simulink model "model2_smartDecision"  (R2020b)
settings: Solver=FixedStepDiscrete  StartTime=0.0  StopTime=24*365  FixedStep=0.25  RelTol=1e-3
PreLoadFcn:
  | load SolarArrayData2017
values from neighbouring files (symbols this model uses):
  Ts = 0.25    [SolarArrayData2017.mat]
libraries: simulink x3
settings Model: Creator=yuanlu  LastModifiedBy=yuanlu
settings DataIOCC: ExternalInput=[Time2017, Power2017]  LoadExternalInput=on  SaveFormat=Array

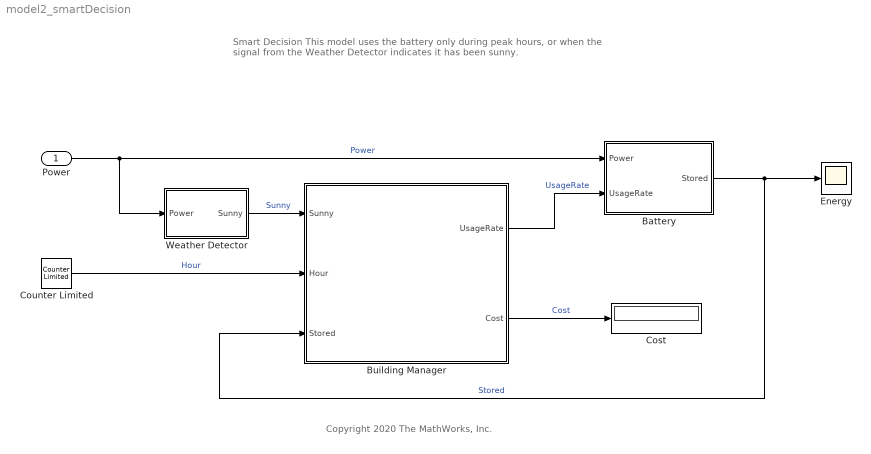
== system model2_smartDecision ==
  note: Smart Decision
      |
      | This model uses the battery only during peak hours, or when the signal from the Weather Detector indicates it has been sunny.
  note: Copyright 2020 The MathWorks, Inc.
  Power : Inport  OutDataTypeStr=double  PortDimensions=1  SampleTime=Ts
  Battery : Subsystem
      settings: PortSchema="{\"entries\":[{\"content\":{\"sides\":[{\"content\":{\"connectorIds\":[\"Out1\"]},\"type\":\"ConnectorPlacement.EquallySpacedRectSide\",\"uuid\":\"59dd599f-b696-4c56-89df-b275042a9a5a\"},{\"content\":{\"connectorIds\":[\"In1\",\"In2\"],\"side\":\"RIGHT\"},\"type\":\"ConnectorPlacement.EquallySpacedRectSide\",\"uuid\":\"1d44f145-e871-49a8-b378-5950f35f06d2\"},{\"content\":{\"connectorIds\":[],\"side\":\"TOP\"},\"type\":\"ConnectorPlacement.EquallySpacedRectSide\",\"uuid\":\"c2e5aa38-1e8a-44d9-a957-b66bd8298b0c\"}]},\"type\":\"ConnectorPlacement.EquallySpacedConnector\",\"uuid\":\"d1e4dde8-4f57-4dd9-974e-75c5ff0ff283\"}],\"packageUris\":[\"http://schema.mathworks.com/mf0/Connector/19700101\"],\"version\":\"1.0\"}"
  Building Manager : Stateflow chart  TreatAsAtomicUnit=on
  Cost : Display
      settings: Format=bank
  Counter Limited : simulink/Sources/Counter Limited  uplimit=23  tsamp=1
  Energy : Scope
  Weather Detector : Subsystem
  wires:
  Power/1 -> Battery/1(Power), Weather Detector/1(Power)  "Power"
  Weather Detector/1(Sunny) -> Building Manager/1(Sunny)  "Sunny"
  Building Manager/2(Cost) -> Cost/1  "Cost"
  Counter Limited/1 -> Building Manager/2(Hour)  "Hour"
  Building Manager/1(UsageRate) -> Battery/2(UsageRate)  "UsageRate"
  Battery/1(Stored) -> Energy/1, Building Manager/3(Stored)  "Stored"

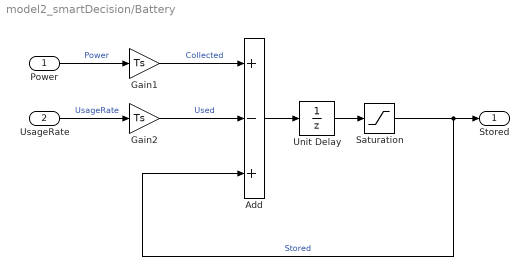
== system model2_smartDecision/Battery ==
  Power : Inport
  UsageRate : Inport  Port=2
  Add : Sum  Inputs=+-+
  Gain1 : Gain  Gain=Ts
  Gain2 : Gain  Gain=Ts
  Saturation : Saturate  UpperLimit=3000  LowerLimit=-inf
  Unit Delay : UnitDelay  SampleTime=Ts  HasFrameUpgradeWarning=on
  Stored : Outport
  wires:
  Add/1 -> Unit Delay/1
  Power/1 -> Gain1/1  "Power"
  Unit Delay/1 -> Saturation/1
  Gain1/1 -> Add/1  "Collected"
  UsageRate/1 -> Gain2/1  "UsageRate"
  Gain2/1 -> Add/2  "Used"
  Saturation/1 -> Add/3, Stored/1  "Stored"

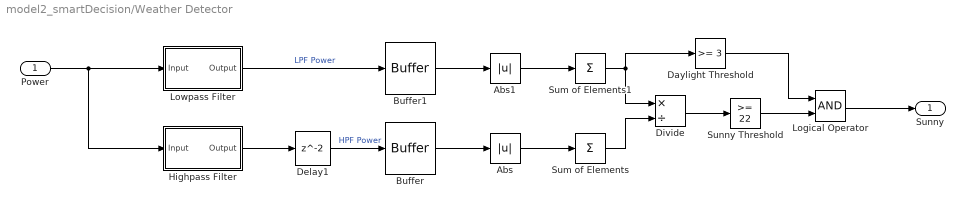
== system model2_smartDecision/Weather Detector ==
  Power : Inport
  Abs : Abs
  Abs1 : Abs
  Buffer : Buffer  N=12  OutputFrames=off
  Buffer1 : Buffer  N=12  OutputFrames=off
  Daylight Threshold : simulink/Logic and Bit Operations/Compare To Constant  relop=>=  const=3  OutDataTypeStr=boolean
  Delay1 : Delay
  Divide : Product  Inputs=*/
  Highpass Filter : Subsystem  Tag=FilterWizardSubSystem
      settings: ErrorFcn=dspFilterRealizedInBasicElemsAlgLoopErrFcnCallback
  Logical Operator : Logic  AllPortsSameDT=off  OutDataTypeStr=boolean
  Lowpass Filter : Subsystem  Tag=FilterWizardSubSystem
      settings: ErrorFcn=dspFilterRealizedInBasicElemsAlgLoopErrFcnCallback
  Sum of Elements : Sum  Inputs=+
  Sum of Elements1 : Sum  Inputs=+
  Sunny Threshold : simulink/Logic and Bit Operations/Compare To Constant  relop=>=  const=22  OutDataTypeStr=boolean
  Sunny : Outport
  wires:
  Divide/1 -> Sunny Threshold/1
  Sum of Elements1/1 -> Divide/1, Daylight Threshold/1
  Sum of Elements/1 -> Divide/2
  Abs/1 -> Sum of Elements/1
  Buffer1/1 -> Abs1/1
  Power/1 -> Highpass Filter/1(Input), Lowpass Filter/1(Input)
  Logical Operator/1 -> Sunny/1
  Daylight Threshold/1 -> Logical Operator/1
  Lowpass Filter/1(Output) -> Buffer1/1  "LPF Power"
  Highpass Filter/1(Output) -> Delay1/1
  Sunny Threshold/1 -> Logical Operator/2
  Delay1/1 -> Buffer/1  "HPF Power"
  Buffer/1 -> Abs/1
  Abs1/1 -> Sum of Elements1/1

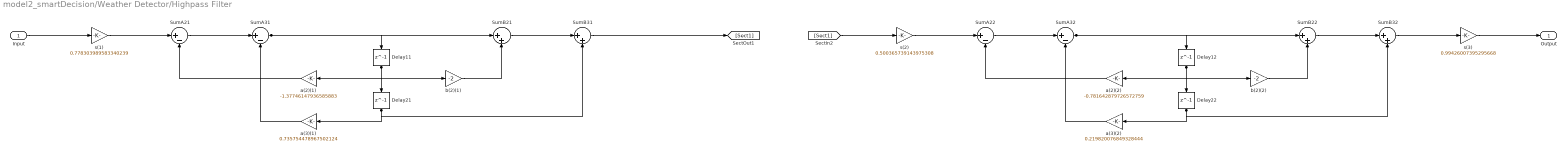
== system model2_smartDecision/Weather Detector/Highpass Filter ==
  Input : Inport
  Delay{11..12,21..22} (4 alike) : Delay  DelayLength=1  InitialCondition=0
  SumA{21..22,31..32} (4 alike) : Sum  Inputs=|+-  RndMeth=Nearest  SaturateOnIntegerOverflow=on  OutDataTypeStr=Inherit: Same as first input
  SumB{21..22,31..32} (4 alike) : Sum  Inputs=|++  RndMeth=Nearest  SaturateOnIntegerOverflow=on  OutDataTypeStr=Inherit: Same as first input
  a(2)(1) : Gain  Gain=-1.37746147936585883  ParamDataTypeStr=double  RndMeth=Nearest  SaturateOnIntegerOverflow=on  OutDataTypeStr=Inherit: Same as input
  a(2)(2) : Gain  Gain=-0.781642879726572759  ParamDataTypeStr=double  RndMeth=Nearest  SaturateOnIntegerOverflow=on  OutDataTypeStr=Inherit: Same as input
  a(3)(1) : Gain  Gain=0.735754478967502124  ParamDataTypeStr=double  RndMeth=Nearest  SaturateOnIntegerOverflow=on  OutDataTypeStr=Inherit: Same as input
  a(3)(2) : Gain  Gain=0.219820076849328444  ParamDataTypeStr=double  RndMeth=Nearest  SaturateOnIntegerOverflow=on  OutDataTypeStr=Inherit: Same as input
  b(2)(1) : Gain  Gain=-2  ParamDataTypeStr=double  RndMeth=Nearest  SaturateOnIntegerOverflow=on  OutDataTypeStr=Inherit: Same as input
  b(2)(2) : Gain  Gain=-2  ParamDataTypeStr=double  RndMeth=Nearest  SaturateOnIntegerOverflow=on  OutDataTypeStr=Inherit: Same as input
  s(1) : Gain  Gain=0.778303989583340239  ParamDataTypeStr=double  RndMeth=Nearest  SaturateOnIntegerOverflow=on  OutDataTypeStr=Inherit: Same as input
  s(2) : Gain  Gain=0.500365739143975308  ParamDataTypeStr=double  RndMeth=Nearest  SaturateOnIntegerOverflow=on  OutDataTypeStr=Inherit: Same as input
  s(3) : Gain  Gain=0.99426007395295668  ParamDataTypeStr=double  RndMeth=Nearest  SaturateOnIntegerOverflow=on  OutDataTypeStr=Inherit: Same as input
  Output : Outport
  wires:
  Input/1 -> s(1)/1
  s(1)/1 -> SumA21/1
  SumA21/1 -> SumA31/1
  SumA31/1 -> SumB21/1, Delay11/1
  SumB21/1 -> SumB31/1
  SumB31/1 -> [Sect1]
  a(2)(1)/1 -> SumA21/2
  Delay11/1 -> a(2)(1)/1, b(2)(1)/1, Delay21/1
  b(2)(1)/1 -> SumB21/2
  a(3)(1)/1 -> SumA31/2
  Delay21/1 -> a(3)(1)/1, SumB31/2
  [Sect1] -> s(2)/1
  s(2)/1 -> SumA22/1
  SumA22/1 -> SumA32/1
  SumA32/1 -> SumB22/1, Delay12/1
  SumB22/1 -> SumB32/1
  SumB32/1 -> s(3)/1
  a(2)(2)/1 -> SumA22/2
  Delay12/1 -> a(2)(2)/1, b(2)(2)/1, Delay22/1
  b(2)(2)/1 -> SumB22/2
  a(3)(2)/1 -> SumA32/2
  Delay22/1 -> a(3)(2)/1, SumB32/2
  s(3)/1 -> Output/1

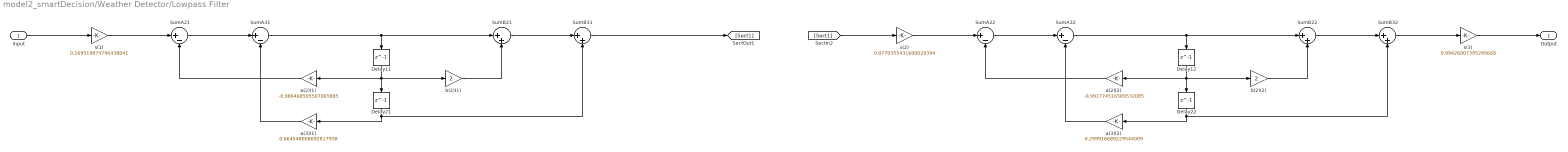
== system model2_smartDecision/Weather Detector/Lowpass Filter ==
  Input : Inport
  Delay{11..12,21..22} (4 alike) : Delay  DelayLength=1  InitialCondition=0
  SumA{21..22,31..32} (4 alike) : Sum  Inputs=|+-  RndMeth=Nearest  SaturateOnIntegerOverflow=on  OutDataTypeStr=Inherit: Same as first input
  SumB{21..22,31..32} (4 alike) : Sum  Inputs=|++  RndMeth=Nearest  SaturateOnIntegerOverflow=on  OutDataTypeStr=Inherit: Same as first input
  a(2)(1) : Gain  Gain=-0.986468505507065885  ParamDataTypeStr=double  RndMeth=Nearest  SaturateOnIntegerOverflow=on  OutDataTypeStr=Inherit: Same as input
  a(2)(2) : Gain  Gain=-0.991774516589532085  ParamDataTypeStr=double  RndMeth=Nearest  SaturateOnIntegerOverflow=on  OutDataTypeStr=Inherit: Same as input
  a(3)(1) : Gain  Gain=0.664548008692817938  ParamDataTypeStr=double  RndMeth=Nearest  SaturateOnIntegerOverflow=on  OutDataTypeStr=Inherit: Same as input
  a(3)(2) : Gain  Gain=0.299916689229544009  ParamDataTypeStr=double  RndMeth=Nearest  SaturateOnIntegerOverflow=on  OutDataTypeStr=Inherit: Same as input
  b(2)(1) : Gain  Gain=2  ParamDataTypeStr=double  RndMeth=Nearest  SaturateOnIntegerOverflow=on  OutDataTypeStr=Inherit: Same as input
  b(2)(2) : Gain  Gain=2  ParamDataTypeStr=double  RndMeth=Nearest  SaturateOnIntegerOverflow=on  OutDataTypeStr=Inherit: Same as input
  s(1) : Gain  Gain=0.169519875796438041  ParamDataTypeStr=double  RndMeth=Nearest  SaturateOnIntegerOverflow=on  OutDataTypeStr=Inherit: Same as input
  s(2) : Gain  Gain=0.0770355431600029394  ParamDataTypeStr=double  RndMeth=Nearest  SaturateOnIntegerOverflow=on  OutDataTypeStr=Inherit: Same as input
  s(3) : Gain  Gain=0.99426007395295668  ParamDataTypeStr=double  RndMeth=Nearest  SaturateOnIntegerOverflow=on  OutDataTypeStr=Inherit: Same as input
  Output : Outport
  wires:
  Input/1 -> s(1)/1
  s(1)/1 -> SumA21/1
  SumA21/1 -> SumA31/1
  SumA31/1 -> SumB21/1, Delay11/1
  SumB21/1 -> SumB31/1
  SumB31/1 -> [Sect1]
  a(2)(1)/1 -> SumA21/2
  Delay11/1 -> a(2)(1)/1, b(2)(1)/1, Delay21/1
  b(2)(1)/1 -> SumB21/2
  a(3)(1)/1 -> SumA31/2
  Delay21/1 -> a(3)(1)/1, SumB31/2
  [Sect1] -> s(2)/1
  s(2)/1 -> SumA22/1
  SumA22/1 -> SumA32/1
  SumA32/1 -> SumB22/1, Delay12/1
  SumB22/1 -> SumB32/1
  SumB32/1 -> s(3)/1
  a(2)(2)/1 -> SumA22/2
  Delay12/1 -> a(2)(2)/1, b(2)(2)/1, Delay22/1
  b(2)(2)/1 -> SumB22/2
  a(3)(2)/1 -> SumA32/2
  Delay22/1 -> a(3)(2)/1, SumB32/2
  s(3)/1 -> Output/1

== stateflow chart model2_smartDecision/Building Manager ==
  state Time [parallel]
    settings: executionOrder=1
    state OffPeak
    state Peak
    (default) -> OffPeak
    OffPeak -> Peak : [Hour >= 12 && Hour < 18]
    Peak -> OffPeak : [Hour >= 18]
  state EnergyManager [parallel]
    settings: executionOrder=2
    state UseGrid
      (default) -> (junction 164)
      UseGrid -> (junction 164) [order 1]
      (junction 164) -> (junction 155) [order 1] : [in(Time.Peak)]
      (junction 164) -> (junction 161) [order 2] : {Cost = Cost + 10;}
      (junction 155) -> (junction 157) : {Cost = Cost + 15;}
      (junction 157) -> (junction 161)
    state UseBattery
      entry:
      UsageRate = 200;
      exit:
      UsageRate = 0;
    (default) -> UseGrid : {Cost = 0;}
    UseGrid -> (junction 168) [order 1] : [Stored > 50]
    (junction 168) -> (junction 169) [order 1] : [in(Time.Peak)]
    (junction 168) -> (junction 174) [order 2]
    (junction 169) -> UseBattery
    (junction 174) -> UseBattery : [in(Time.OffPeak) && Sunny]
    UseBattery -> UseGrid : [Stored < 50]
  data: UsageRate output; Cost output; Sunny input; Hour input; Stored input =0
